simulink model "VTOLAutopilotController"  (R2025a)
settings: configuration reference "VTOLConfiguration" (kept outside this file)
undefined symbols (not defined in the file): Back_Transition_Rate, const, control, controlParams, ControlSampleTime, CriticalTiltAngle, DiscIntNeverNeededParam, dspblkCoreblockFVToolHelper, Fading_time, flightState, FSState, FWControlParams, FWTrimSpeed, gcbh, HoverMission, ReferenceFilterDen, ReferenceFilterNum, tilt_max, tiltIni, TransitioncontrolGains, uavParam, uavParams, VTOLcontrolGains, w_trim, WindDownRate
libraries: simulink x43, slpidlib x35, uavalgslib x7, simulink_extras x1
(part 4 of 8)

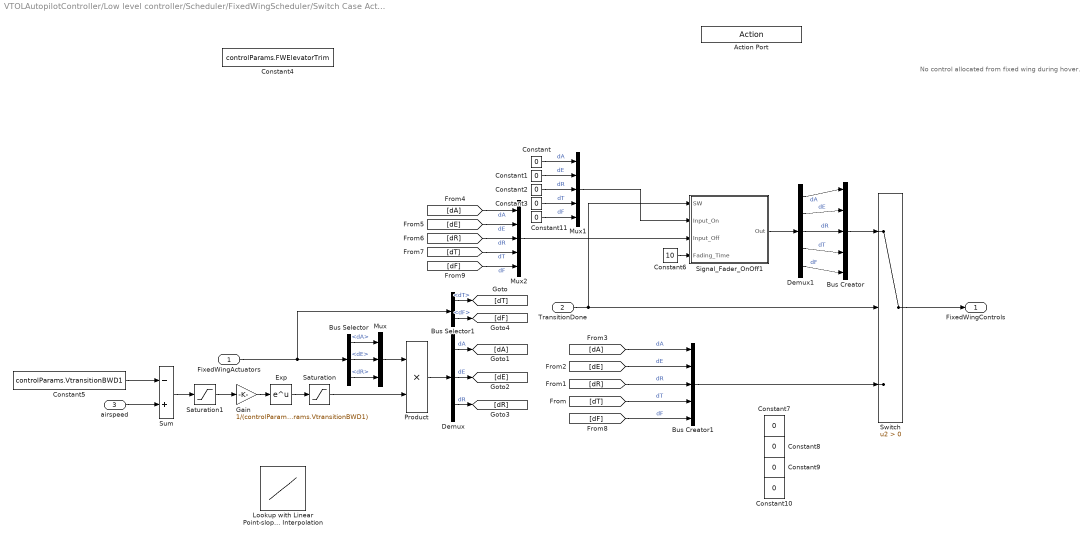
== system VTOLAutopilotController/Low level controller/Scheduler/FixedWingScheduler/Switch Case Action Subsystem3 ==
  note: No control allocated from fixed wing during hover.
  FixedWingActuators : Inport  OutDataTypeStr=Bus: FixedWingCtrlBus
  TransitionDone : Inport  Port=2
  airspeed : Inport  Port=3
  Action Port : ActionPort  ActionPortLabel=case [ BackTransition ]:
  Bus Creator : BusCreator  Inputs=5
  Bus Creator1 : BusCreator  Inputs=5  OutDataTypeStr=Bus: FixedWingCtrlBus
  Bus Selector : BusSelector  OutputSignals=dA,dE,dR
  Bus Selector1 : BusSelector  OutputSignals=dT,dF
  Constant{,1..3,7..11} (9 alike) : Constant  Value=0
  Constant4 : Constant  Value=controlParams.FWElevatorTrim
  Constant5 : Constant  Value=controlParams.VtransitionBWD1
  Constant6 : Constant  Value=10
  Demux : Demux  Outputs=3
  Demux1 : Demux  Outputs=5
  Exp : Math
  Gain : Gain  Gain=1/(controlParams.VtransitionBWD2-controlParams.VtransitionBWD1)
  Lookup with Linear Point-slope Interpolation : Lookup_n-D  NumberOfTableDimensions=1  BreakpointsForDimension1=[10 20 30 40 50 60]*const.kts2mps  Table=[1.0 1.0 0.8 0.5 0.1]  InternalRulePriority=Speed  RndMeth=Simplest
  Mux : Mux  Inputs=3
  Mux1 : Mux  Inputs=5
  Mux2 : Mux  Inputs=5
  Product : Product
  Saturation : Saturate  UpperLimit=1  LowerLimit=0
  Saturation1 : Saturate  UpperLimit=0  LowerLimit=controlParams.VtransitionBWD2-controlParams.VtransitionBWD1
  Signal_Fader_OnOff1 : Subsystem
  Sum : Sum  Inputs=-+
  Switch : Switch  Criteria=u2 > Threshold  SaturateOnIntegerOverflow=off  InputSameDT=off
  FixedWingControls : Outport  OutDataTypeStr=Bus: FixedWingCtrlBus
  wires:
  Bus Selector1/1 -> [dT]  "<dT>"
  Saturation1/1 -> Gain/1
  Demux/2 -> [dE]  "dE"
  Mux/1 -> Product/1
  Bus Selector/1 -> Mux/1  "<dA>"
  Bus Selector/2 -> Mux/2  "<dE>"
  Sum/1 -> Saturation1/1
  Product/1 -> Demux/1
  Constant5/1 -> Sum/1
  Saturation/1 -> Product/2
  Exp/1 -> Saturation/1
  Bus Selector/3 -> Mux/3  "<dR>"
  TransitionDone/1 -> Signal_Fader_OnOff1/1(SW), Switch/2
  FixedWingActuators/1 -> Bus Selector1/1, Bus Selector/1
  Demux/1 -> [dA]  "dA"
  airspeed/1 -> Sum/2
  Demux/3 -> [dR]  "dR"
  Gain/1 -> Exp/1
  Switch/1 -> FixedWingControls/1
  Constant6/1 -> Signal_Fader_OnOff1/4(Fading_Time)
  Bus Creator/1 -> Switch/1
  Demux1/3 -> Bus Creator/3  "dR"
  Demux1/2 -> Bus Creator/2  "dE"
  Demux1/4 -> Bus Creator/4  "dT"
  Demux1/1 -> Bus Creator/1  "dA"
  Signal_Fader_OnOff1/1(Out) -> Demux1/1
  Constant/1 -> Mux1/1  "dA"
  Constant1/1 -> Mux1/2  "dE"
  Constant2/1 -> Mux1/3  "dR"
  Constant3/1 -> Mux1/4  "dT"
  [dA] -> Mux2/1  "dA"
  [dE] -> Mux2/2  "dE"
  [dR] -> Mux2/3  "dR"
  [dT] -> Mux2/4  "dT"
  Mux1/1 -> Signal_Fader_OnOff1/2(Input_On)
  Mux2/1 -> Signal_Fader_OnOff1/3(Input_Off)
  Bus Creator1/1 -> Switch/3
  [dA] -> Bus Creator1/1  "dA"
  [dE] -> Bus Creator1/2  "dE"
  [dR] -> Bus Creator1/3  "dR"
  [dT] -> Bus Creator1/4  "dT"
  Constant11/1 -> Mux1/5  "dF"
  Bus Selector1/2 -> [dF]  "<dF>"
  [dF] -> Mux2/5  "dF"
  Demux1/5 -> Bus Creator/5  "dF"
  [dF] -> Bus Creator1/5  "dF"

== system VTOLAutopilotController/Low level controller/Scheduler/Subsystem/Actuator To Voltage ==
  note: #2, 25/05/20, MH, Fixed
      | The rotor rotational speed command should be
      | normalized to [rad/s].Previously, division by 2PI
      | was omitted in the command block,
      | while the 'Rotor Assembly' block multiplies
      | the input by 2PI, leading to increased gains.
  Motor Commands : Inport
  Bus Creator : BusCreator  Inputs=6  OutDataTypeStr=Bus: RotorCtrlBus
  Bus Selector : BusSelector  OutputSignals=w1,w2,w3,w4,Tilt1,Tilt2
  Gain{,1..2,4} (4 alike) : Gain  Gain=1/(uavParams.motor.RPMMAX/60)
  Gain3 : Gain  Gain=1/(pi/2)
  Gain5 : Gain  Gain=1/(pi/2)
  Gain{6..9} (4 alike) : Gain  Gain=1/(2*pi)
  Saturation{,1..3} (4 alike) : Saturate  UpperLimit=controlParams.maxPWM  LowerLimit=controlParams.minPWM
  Saturation4 : Saturate  UpperLimit=1  LowerLimit=0
  Saturation5 : Saturate  UpperLimit=1  LowerLimit=0
  To PWM : Outport
  wires:
  Motor Commands/1 -> Bus Selector/1
  Bus Selector/1 -> Gain/1  "<w1>"
  Bus Selector/3 -> Gain1/1  "<w3>"
  Bus Selector/2 -> Gain4/1  "<w2>"
  Bus Selector/4 -> Gain2/1  "<w4>"
  Bus Selector/5 -> Gain3/1  "<Tilt1>"
  Bus Selector/6 -> Gain5/1  "<Tilt2>"
  Gain/1 -> Gain6/1  "w1"
  Gain4/1 -> Gain7/1  "w2"
  Gain1/1 -> Gain8/1  "w3"
  Gain2/1 -> Gain9/1  "w4"
  Gain3/1 -> Saturation4/1
  Gain5/1 -> Saturation5/1
  Bus Creator/1 -> To PWM/1
  Gain6/1 -> Saturation/1
  Gain7/1 -> Saturation1/1
  Gain8/1 -> Saturation2/1
  Gain9/1 -> Saturation3/1
  Saturation/1 -> Bus Creator/1  "w1"
  Saturation1/1 -> Bus Creator/2  "w2"
  Saturation2/1 -> Bus Creator/3  "w3"
  Saturation3/1 -> Bus Creator/4  "w4"
  Saturation4/1 -> Bus Creator/5  "Tilt1"
  Saturation5/1 -> Bus Creator/6  "Tilt2"

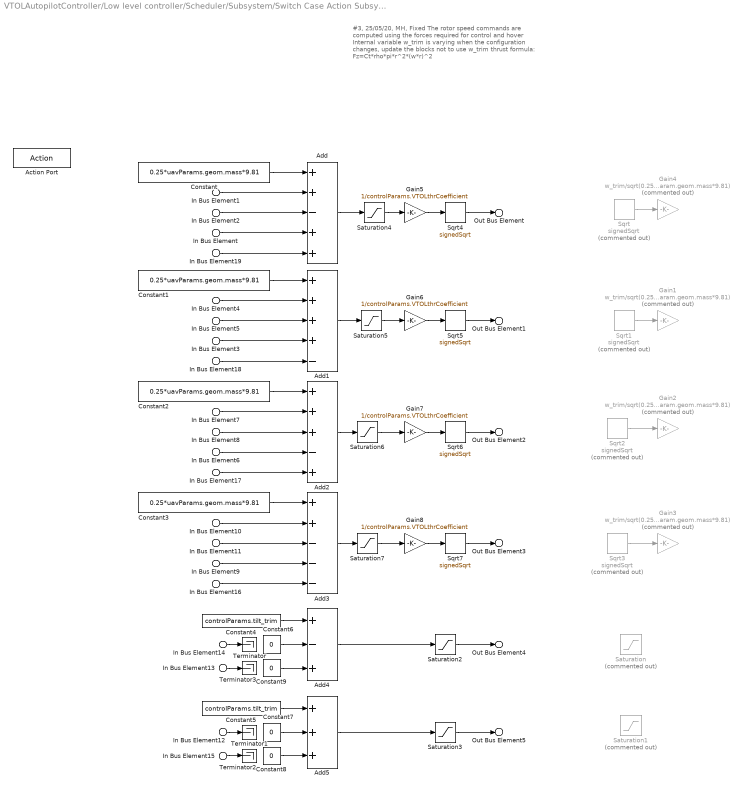
== system VTOLAutopilotController/Low level controller/Scheduler/Subsystem/Switch Case Action Subsystem ==
  note: #3, 25/05/20, MH, Fixed
      | The rotor speed commands are computed using
      | the forces required for control and hover
      | Internal variable w_trim is varying when the
      | configuration changes, update the blocks not to
      | use w_trim
      | thrust formula: Fz=Ct*rho*pi*r^2*(w*r)^2
  In Bus Element{,3,6,9} (4 alike) : Inport  PortName=MixerCommands  Element=w_theta
  In Bus Element{1,4,7,10} (4 alike) : Inport  PortName=MixerCommands  Element=w_z
  In Bus Element{2,5,8,11} (4 alike) : Inport  PortName=MixerCommands  Element=w_phi
  In Bus Element{12,14,16..19} (6 alike) : Inport  PortName=MixerCommands  Element=w_psi
  In Bus Element13 : Inport  PortName=MixerCommands  Element=w_tilt
  In Bus Element15 : Inport  PortName=MixerCommands  Element=w_tilt
  Action Port : ActionPort  ActionPortLabel=case [ Hover ]:
  Add : Sum  Inputs=++-++
  Add1 : Sum  Inputs=++++-
  Add2 : Sum  Inputs=+++-+
  Add3 : Sum  Inputs=++---
  Add4 : Sum  Inputs=+-+
  Add5 : Sum  Inputs=+++
  Constant{,1..3} (4 alike) : Constant  Value=0.25*uavParams.geom.mass*9.81
  Constant4 : Constant  Value=controlParams.tilt_trim
  Constant5 : Constant  Value=controlParams.tilt_trim
  Constant{6..9} (4 alike) : Constant  Value=0
  Gain{1..4} (4 alike) : Gain  Commented=on  Gain=w_trim/sqrt(0.25*uavParam.geom.mass*9.81)
  Gain{5..8} (4 alike) : Gain  Gain=1/controlParams.VTOLthrCoefficient
  Saturation : Saturate  Commented=on  UpperLimit=tilt_max  LowerLimit=-tilt_max
  Saturation1 : Saturate  Commented=on  UpperLimit=tilt_max  LowerLimit=-tilt_max
  Saturation2 : Saturate  UpperLimit=tilt_max  LowerLimit=-tilt_max
  Saturation3 : Saturate  UpperLimit=tilt_max  LowerLimit=-tilt_max
  Saturation{4..7} (4 alike) : Saturate  UpperLimit=inf  LowerLimit=0
  Sqrt{,1..3} (4 alike) : Sqrt  Commented=on  Operator=signedSqrt
  Sqrt{4..7} (4 alike) : Sqrt  Operator=signedSqrt
  Terminator{,1..3} (4 alike) : Terminator
  Out Bus Element : Outport  PortName=Actuator  Element=w1
  Out Bus Element1 : Outport  PortName=Actuator  Element=w2
  Out Bus Element2 : Outport  PortName=Actuator  Element=w3
  Out Bus Element3 : Outport  PortName=Actuator  Element=w4
  Out Bus Element4 : Outport  PortName=Actuator  Element=Tilt1
  Out Bus Element5 : Outport  PortName=Actuator  Element=Tilt2
  wires:
  Constant5/1 -> Add5/1
  Constant2/1 -> Add2/1
  Constant1/1 -> Add1/1
  Constant4/1 -> Add4/1
  Constant/1 -> Add/1
  Constant3/1 -> Add3/1
  Add/1 -> Saturation4/1
  Add1/1 -> Saturation5/1
  Add2/1 -> Saturation6/1
  Add3/1 -> Saturation7/1
  Saturation2/1 -> Out Bus Element4/1
  Add4/1 -> Saturation2/1
  Add5/1 -> Saturation3/1
  Saturation3/1 -> Out Bus Element5/1
  Saturation4/1 -> Gain5/1
  Saturation5/1 -> Gain6/1
  Saturation6/1 -> Gain7/1
  Saturation7/1 -> Gain8/1
  Sqrt4/1 -> Out Bus Element/1
  Sqrt5/1 -> Out Bus Element1/1
  Sqrt6/1 -> Out Bus Element2/1
  Sqrt7/1 -> Out Bus Element3/1
  In Bus Element2/1 -> Add/3
  In Bus Element/1 -> Add/4
  In Bus Element5/1 -> Add1/3
  In Bus Element3/1 -> Add1/4
  In Bus Element8/1 -> Add2/3
  In Bus Element11/1 -> Add3/3
  In Bus Element9/1 -> Add3/4
  In Bus Element6/1 -> Add2/4
  Sqrt/1 -> Gain4/1
  Sqrt3/1 -> Gain3/1
  Sqrt2/1 -> Gain2/1
  Sqrt1/1 -> Gain1/1
  Gain5/1 -> Sqrt4/1
  Gain6/1 -> Sqrt5/1
  Gain7/1 -> Sqrt6/1
  Gain8/1 -> Sqrt7/1
  In Bus Element1/1 -> Add/2
  In Bus Element4/1 -> Add1/2
  In Bus Element7/1 -> Add2/2
  In Bus Element10/1 -> Add3/2
  In Bus Element19/1 -> Add/5
  In Bus Element16/1 -> Add3/5
  In Bus Element17/1 -> Add2/5
  In Bus Element18/1 -> Add1/5
  In Bus Element14/1 -> Terminator/1
  In Bus Element12/1 -> Terminator1/1
  Constant6/1 -> Add4/2
  Constant7/1 -> Add5/2
  Constant8/1 -> Add5/3
  In Bus Element15/1 -> Terminator2/1
  Constant9/1 -> Add4/3
  In Bus Element13/1 -> Terminator3/1

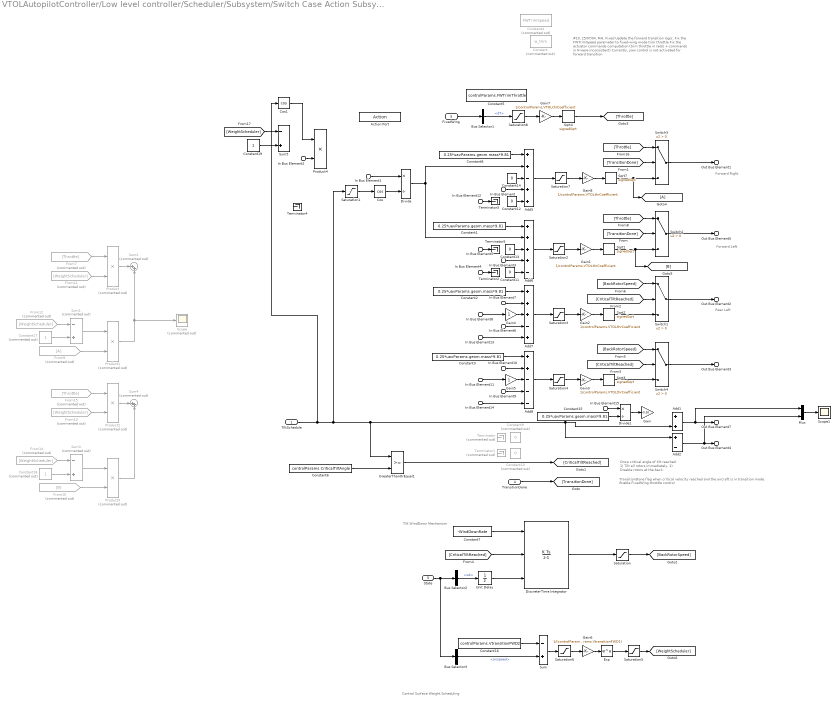
== system VTOLAutopilotController/Low level controller/Scheduler/Subsystem/Switch Case Action Subsystem1 ==
  note: Tilt WindDown Mechanism
  note: Once critical angle of tilt reached.
      | 1) Tilt all rotors immediately.
      | 2) Disable rotors at the back.
  note: TransitionDone flag when critical velocity reached and the aircraft is in transition mode.
      | Enable FixedWing throttle control
  note: #10, 25/07/04, MH, Fixed
      | Update the forward transition logic.
      | Fix the FWTrimSpeed parameter to fixed-wing
      | mode trim throttle
      | Fix the actuator commands computation
      | (trim throttle in rad/s + commands in N were
      | inconsistent)
      | Currently, yaw control is not activated for
      | forward transition
  note: Rear Left
  note: Forward Right
  note: Forward Left
  note: Control Surface Weight Scheduling
  TiltSchedule : Inport
  In Bus Element{,3,6,9} (4 alike) : Inport  Port=2  PortName=MixerCommands  Element=w_theta
  In Bus Element1 : Inport  Port=2  PortName=MixerCommands  Element=w_z
  In Bus Element7 : Inport  Port=2  PortName=MixerCommands  Element=w_z
  In Bus Element10 : Inport  Port=2  PortName=MixerCommands  Element=w_z
  In Bus Element{2,5,8,11} (4 alike) : Inport  Port=2  PortName=MixerCommands  Element=w_phi
  In Bus Element{4,12..15} (5 alike) : Inport  Port=2  PortName=MixerCommands  Element=w_psi
  FixedWing : Inport  Port=3
  TransitionDone : Inport  Port=4
  State : Inport  Port=5
  Action Port : ActionPort  ActionPortLabel=case [ Transition ]:
  Add1 : Sum
  Add2 : Sum  Inputs=+-
  Add5 : Sum  Inputs=++-++
  Add6 : Sum  Inputs=++++-
  Add7 : Sum  Inputs=+++-+
  Add8 : Sum  Inputs=++---
  Bus Selector1 : BusSelector  OutputSignals=dT
  Bus Selector2 : BusSelector  OutputSignals=RotorParameters.w4
  Bus Selector3 : BusSelector  OutputSignals=airspeed
  Constant : Constant  Commented=on  Value=w_trim
  Constant{1..3,8,15} (5 alike) : Constant  Value=0.25*uavParams.geom.mass*9.81
  Constant10 : Constant  Commented=on  Value=0
  Constant{11..14} (4 alike) : Constant  Value=0
  Constant16 : Constant  Value=controlParams.VtransitionFWD2
  Constant17 : Constant  Commented=on
  Constant18 : Constant  Commented=on
  Constant19 : Constant
  Constant4 : Constant  Commented=on  Value=FWTrimSpeed
  Constant5 : Constant  Value=controlParams.FWTrimThrottle
  Constant6 : Constant  Value=controlParams.CriticalTiltAngle
  Constant7 : Constant  Value=-WindDownRate
  Constant9 : Constant  Commented=on  Value=0
  Cos : Trigonometry  Operator=cos
  Cos1 : Trigonometry  Operator=cos
  Discrete-Time Integrator : DiscreteIntegrator  ExternalReset=either  InitialConditionSource=external  SampleTime=0.005  ICPrevOutput=DiscIntNeverNeededParam  ICPrevScaledInput=DiscIntNeverNeededParam
  Divide : Product  Inputs=*/
  Divide1 : Product  Inputs=*/
  Exp : Math
  From10 : From  Commented=on  GotoTag=B
  From{11..14} (4 alike) : From  Commented=on  GotoTag=WeightScheduler
  From15 : From  Commented=on  GotoTag=Throttle
  From7 : From  Commented=on  GotoTag=Throttle
  From9 : From  Commented=on
  Gain : Gain  Gain=-0.30
  Gain{1..3,7..8} (5 alike) : Gain  Gain=1/controlParams.VTOLthrCoefficient
  Gain4 : Gain
  Gain5 : Gain
  Gain6 : Gain  Gain=1/(controlParams.VtransitionFWD2-controlParams.VtransitionFWD1)
  Goto4 : Goto
  GreaterThanOrEqual1 : RelationalOperator  OutDataTypeStr=boolean  RndMeth=Simplest  InputSameDT=off
  Mux : Mux  Inputs=2
  Product{,1..3} (4 alike) : Product  Commented=on
  Product4 : Product
  Saturation : Saturate  UpperLimit=Inf  LowerLimit=0
  Saturation1 : Saturate  UpperLimit=CriticalTiltAngle  LowerLimit=-CriticalTiltAngle
  Saturation{2..4,7..8} (5 alike) : Saturate  UpperLimit=inf  LowerLimit=0
  Saturation5 : Saturate  UpperLimit=1  LowerLimit=0
  Saturation6 : Saturate  UpperLimit=0  LowerLimit=controlParams.VtransitionFWD1-controlParams.VtransitionFWD2
  Scope : Scope  Commented=on
      settings: ActiveDisplayYMinimum=-118.86543  ActiveDisplayYMaximum=1069.7889
  Scope1 : Scope
      settings: ActiveDisplayYMinimum=-0.19635  ActiveDisplayYMaximum=1.76715  DataLoggingVariableName=ScopeData3
  Sqrt{1..4,7} (5 alike) : Sqrt  Operator=signedSqrt
  Sum : Sum  Inputs=-+
  Sum1 : Sum  Commented=on  Inputs=-+
  Sum2 : Sum  Commented=on  Inputs=|++
  Sum3 : Sum  Commented=on  Inputs=-+
  Sum4 : Sum  Commented=on  Inputs=|++
  Sum5 : Sum  Inputs=-+
  Switch{1..4} (4 alike) : Switch  Criteria=u2 > Threshold  SaturateOnIntegerOverflow=off  InputSameDT=off
  Terminator : Terminator  Commented=on
  Terminator1 : Terminator  Commented=on
  Terminator{2..5} (4 alike) : Terminator
  Unit Delay : UnitDelay  SampleTime=-1  HasFrameUpgradeWarning=on
  Out Bus Element1 : Outport  PortName=Actuator  Element=w1
  Out Bus Element5 : Outport  PortName=Actuator  Element=w2
  Out Bus Element2 : Outport  PortName=Actuator  Element=w3
  Out Bus Element3 : Outport  PortName=Actuator  Element=w4
  Out Bus Element7 : Outport  PortName=Actuator  Element=Tilt1
  Out Bus Element4 : Outport  PortName=Actuator  Element=Tilt2
  wires:
  TiltSchedule/1 -> Cos1/1, GreaterThanOrEqual1/1, Add2/1, Add1/2, Saturation1/1
  In Bus Element9/1 -> Add8/4
  In Bus Element6/1 -> Add7/4
  Constant3/1 -> Add8/1
  In Bus Element/1 -> Add5/4
  In Bus Element10/1 -> Add8/2
  Constant1/1 -> Add6/1
  In Bus Element3/1 -> Add6/4
  In Bus Element7/1 -> Add7/2
  Constant2/1 -> Add7/1
  FixedWing/1 -> Bus Selector1/1
  [TransitionDone] -> Switch3/2
  Constant6/1 -> GreaterThanOrEqual1/2
  GreaterThanOrEqual1/1 -> [CriticalTiltReached]
  [CriticalTiltReached] -> Switch1/2
  [CriticalTiltReached] -> Switch4/2
  TransitionDone/1 -> [TransitionDone]
  Bus Selector2/1 -> Unit Delay/1  "<w4>"
  Constant7/1 -> Discrete-Time Integrator/1
  [CriticalTiltReached] -> Discrete-Time Integrator/2
  Discrete-Time Integrator/1 -> Saturation/1
  Saturation/1 -> [BackRotorSpeed]
  State/1 -> Bus Selector3/1, Bus Selector2/1
  Unit Delay/1 -> Discrete-Time Integrator/3
  Cos/1 -> Divide/2
  Saturation1/1 -> Cos/1
  In Bus Element1/1 -> Divide/1
  Divide/1 -> Add5/2, Add6/2
  Switch1/1 -> Out Bus Element2/1
  Gain8/1 -> Sqrt7/1
  Saturation7/1 -> Gain8/1
  Constant8/1 -> Add5/1
  Add5/1 -> Saturation7/1
  Sqrt7/1 -> Goto4/1, Switch3/3
  [TransitionDone] -> Switch2/2
  Saturation2/1 -> Gain1/1
  Gain1/1 -> Sqrt1/1
  Add6/1 -> Saturation2/1
  Sqrt1/1 -> [B], Switch2/3
  Gain2/1 -> Sqrt2/1
  Saturation3/1 -> Gain2/1
  Add7/1 -> Saturation3/1
  Gain3/1 -> Sqrt3/1
  Saturation4/1 -> Gain3/1
  Add8/1 -> Saturation4/1
  Constant11/1 -> Add6/5
  Constant12/1 -> Add5/5
  In Bus Element12/1 -> Terminator3/1
  In Bus Element4/1 -> Terminator2/1
  Sqrt3/1 -> Switch4/3
  Switch4/1 -> Out Bus Element3/1
  Sqrt2/1 -> Switch1/3
  [BackRotorSpeed] -> Switch1/1
  [BackRotorSpeed] -> Switch4/1
  In Bus Element2/1 -> Product4/2
  In Bus Element5/1 -> Terminator5/1
  In Bus Element11/1 -> Gain5/1
  In Bus Element8/1 -> Gain4/1
  Add1/1 -> Mux/1, Out Bus Element7/1
  In Bus Element13/1 -> Add7/5
  In Bus Element14/1 -> Add8/5
  In Bus Element15/1 -> Divide1/1
  Constant15/1 -> Divide1/2
  Divide1/1 -> Gain/1
  Add2/1 -> Mux/2, Out Bus Element4/1
  Gain4/1 -> Add7/3
  Gain5/1 -> Add8/3
  Saturation6/1 -> Gain6/1
  Sum/1 -> Saturation6/1
  Product/1 -> Sum2/1
  Constant16/1 -> Sum/1
  Gain6/1 -> Exp/1
  Exp/1 -> Saturation5/1
  From7/1 -> Product/1
  Constant17/1 -> Sum1/2
  Sum1/1 -> Product1/1
  From9/1 -> Product1/2
  Product1/1 -> Scope/1, Sum2/2
  [Throttle] -> Switch2/1
  Saturation5/1 -> [WeightScheduler]
  From11/1 -> Product/2
  From12/1 -> Sum1/1
  Product3/1 -> Sum4/2
  From14/1 -> Sum3/1
  Constant18/1 -> Sum3/2
  Product2/1 -> Sum4/1
  Sum3/1 -> Product3/1
  From10/1 -> Product3/2
  From15/1 -> Product2/1
  From13/1 -> Product2/2
  [Throttle] -> Switch3/1
  Bus Selector3/1 -> Sum/2  "<airspeed>"
  Switch3/1 -> Out Bus Element1/1
  Switch2/1 -> Out Bus Element5/1
  Mux/1 -> Scope1/1
  Constant19/1 -> Sum5/2
  [WeightScheduler] -> Sum5/1
  Cos1/1 -> Product4/1
  Constant13/1 -> Add6/3
  Constant14/1 -> Add5/3
  Saturation8/1 -> Gain7/1
  Gain7/1 -> Sqrt4/1
  Bus Selector1/1 -> Saturation8/1  "<dT>"
  Sqrt4/1 -> [Throttle]

== system VTOLAutopilotController/Low level controller/Scheduler/Subsystem/Switch Case Action Subsystem2 ==
  note: Tilt WindDown Mechanism
  In Bus Element2 : Inport  PortName=FixedWingCtrlBus  Element=dT
  In Bus Element1 : Inport  PortName=FixedWingCtrlBus  Element=dT
  TransitionDone : Inport  Port=2
  State : Inport  Port=3
  Action Port : ActionPort  ActionPortLabel=case [ FixedWing ]:
  Add : Sum  Commented=on
  Add1 : Sum  Commented=on
  Bus Selector2 : BusSelector  OutputSignals=RotorParameters.w4
  Constant : Constant  Commented=on  Value=FWTrimSpeed
  Constant1 : Constant  Value=-WindDownRate
  Constant4 : Constant  Value=pi/2
  Constant5 : Constant  Commented=on  Value=controlParams.FWTrimThrottle
  Constant7 : Constant  Value=pi/2
  Discrete-Time Integrator : DiscreteIntegrator  ExternalReset=rising  InitialConditionSource=external  SampleTime=0.005  ICPrevOutput=DiscIntNeverNeededParam  ICPrevScaledInput=DiscIntNeverNeededParam
  Gain1 : Gain  Gain=1/controlParams.VTOLthrCoefficient
  Gain7 : Gain  Gain=1/controlParams.VTOLthrCoefficient
  Saturation : Saturate  UpperLimit=Inf  LowerLimit=0
  Saturation1 : Saturate  UpperLimit=Inf  LowerLimit=0
  Saturation2 : Saturate  UpperLimit=Inf  LowerLimit=0
  Saturation3 : Saturate  UpperLimit=inf  LowerLimit=0
  Saturation8 : Saturate  UpperLimit=inf  LowerLimit=0
  Sqrt1 : Sqrt  Operator=signedSqrt
  Sqrt4 : Sqrt  Operator=signedSqrt
  Out Bus Element : Outport  PortName=Actuator  Element=w1
  Out Bus Element1 : Outport  PortName=Actuator  Element=w2
  Out Bus Element2 : Outport  PortName=Actuator  Element=w3
  Out Bus Element3 : Outport  PortName=Actuator  Element=w4
  Out Bus Element7 : Outport  PortName=Actuator  Element=Tilt1
  Out Bus Element4 : Outport  PortName=Actuator  Element=Tilt2
  wires:
  Sqrt1/1 -> Saturation1/1
  Constant4/1 -> Out Bus Element4/1
  [BackRotorSpeed] -> Out Bus Element2/1
  Constant7/1 -> Out Bus Element7/1
  In Bus Element2/1 -> Saturation3/1
  Sqrt4/1 -> Saturation/1
  In Bus Element1/1 -> Saturation8/1
  Saturation/1 -> Out Bus Element/1
  Saturation1/1 -> Out Bus Element1/1
  [BackRotorSpeed] -> Out Bus Element3/1
  Bus Selector2/1 -> Discrete-Time Integrator/3  "<w4>"
  Saturation2/1 -> [BackRotorSpeed]
  State/1 -> Bus Selector2/1
  Constant1/1 -> Discrete-Time Integrator/1
  Discrete-Time Integrator/1 -> Saturation2/1
  TransitionDone/1 -> Discrete-Time Integrator/2
  Saturation8/1 -> Gain7/1
  Gain7/1 -> Sqrt4/1
  Saturation3/1 -> Gain1/1
  Gain1/1 -> Sqrt1/1

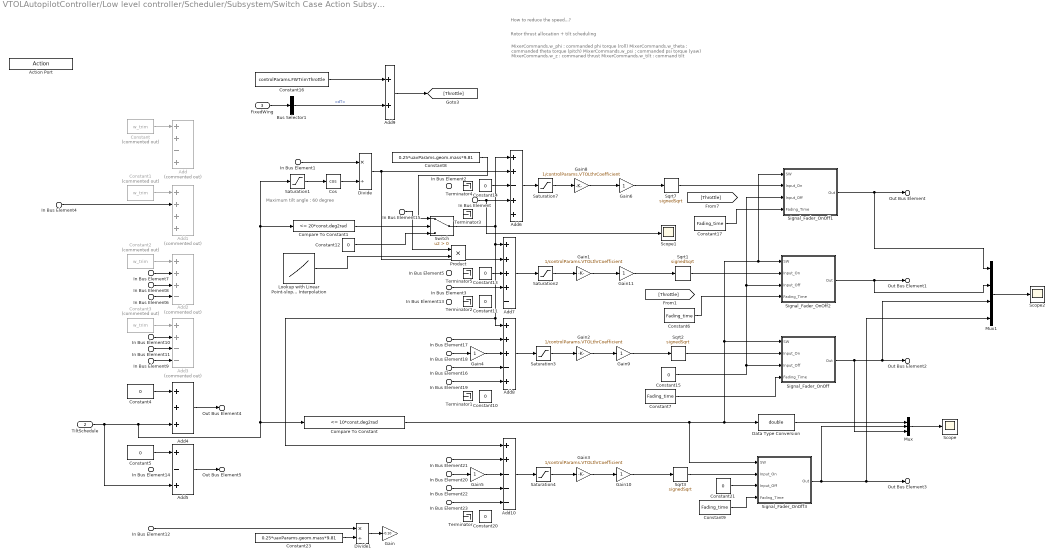
== system VTOLAutopilotController/Low level controller/Scheduler/Subsystem/Switch Case Action Subsystem3 ==
  note: Maximum tilt angle : 60 degree
  note: MixerCommands.w_phi : commanded phi torque (roll)
      | MixerCommands.w_theta : commanded theta torque (pitch)
      | MixerCommands.w_psi : commanded psi torque (yaw)
      | MixerCommands.w_z : commaned thrust
      | MixerCommands.w_tilt : command tilt
  note: Rotor thrust allocation + tilt scheduling
  note: How to reduce the speed...?
  In Bus Element{,3,6,9,16,22} (6 alike) : Inport  PortName=MixerCommands  Element=w_theta
  In Bus Element{1,4,7,10,17,21} (6 alike) : Inport  PortName=MixerCommands  Element=w_z
  In Bus Element{2,5,8,11,18,20} (6 alike) : Inport  PortName=MixerCommands  Element=w_phi
  In Bus Element{12..15,19,23} (6 alike) : Inport  PortName=MixerCommands  Element=w_psi
  TiltSchedule : Inport  Port=2
  FixedWing : Inport  Port=3
  Action Port : ActionPort  ActionPortLabel=case [ BackTransition ]:
  Add : Sum  Commented=on  Inputs=++-+
  Add1 : Sum  Commented=on  Inputs=++++
  Add10 : Sum  Inputs=++---
  Add2 : Sum  Commented=on  Inputs=+++-
  Add3 : Sum  Commented=on  Inputs=++--
  Add4 : Sum  Inputs=+++
  Add5 : Sum  Inputs=+-+
  Add6 : Sum  Inputs=++-++
  Add7 : Sum  Inputs=++++-
  Add8 : Sum  Inputs=+++-+
  Add9 : Sum
  Bus Selector1 : BusSelector  OutputSignals=dT
  Compare To Constant : simulink/Logic and Bit Operations/Compare To Constant  relop=<=  const=10*const.deg2rad  OutDataTypeStr=boolean
  Compare To Constant1 : simulink/Logic and Bit Operations/Compare To Constant  relop=<=  const=20*const.deg2rad  OutDataTypeStr=boolean
  Constant{,1..3} (4 alike) : Constant  Commented=on  Value=w_trim
  Constant{4..5,10..15,20..21} (10 alike) : Constant  Value=0
  Constant16 : Constant  Value=controlParams.FWTrimThrottle
  Constant{6..7,9,17} (4 alike) : Constant  Value=Fading_time
  Constant23 : Constant  Value=0.25*uavParams.geom.mass*9.81
  Constant8 : Constant  Value=0.25*uavParams.geom.mass*9.81
  Cos : Trigonometry  Operator=cos
  Data Type Conversion : DataTypeConversion  OutDataTypeStr=double  SaturateOnIntegerOverflow=off  RndMeth=Floor
  Divide : Product  Inputs=*/
  Divide1 : Product  Inputs=*/
  Gain : Gain  Gain=-0.10
  Gain{1..3,8} (4 alike) : Gain  Gain=1/controlParams.VTOLthrCoefficient
  Gain{4..6,9..11} (6 alike) : Gain
  Lookup with Linear Point-slope Interpolation : Lookup_n-D  NumberOfTableDimensions=1  BreakpointsForDimension1=[10 20 30 40 50 60]*const.kts2mps  Table=[1.0 1.0 0.8 0.5 0.1]  InternalRulePriority=Speed  RndMeth=Simplest
  Mux : Mux  Inputs=3
  Mux1 : Mux
  Product : Product
  Saturation1 : Saturate  UpperLimit=controlParams.CriticalTiltAngle  LowerLimit=-controlParams.CriticalTiltAngle
  Saturation{2..4,7} (4 alike) : Saturate  UpperLimit=inf  LowerLimit=0
  Scope : Scope
      settings: ActiveDisplayYMinimum=-11.37479  ActiveDisplayYMaximum=68.93084  DataLoggingVariableName=ScopeData5
  Scope1 : Scope
      settings: ActiveDisplayYMinimum=-91.47313  ActiveDisplayYMaximum=823.25813
  Scope2 : Scope
      settings: ActiveDisplayYMinimum=325.4581  ActiveDisplayYMaximum=599.86957  DataLoggingVariableName=ScopeData2
  Signal_Fader_OnOff : Subsystem
  Signal_Fader_OnOff1 : Subsystem
  Signal_Fader_OnOff2 : Subsystem
  Signal_Fader_OnOff3 : Subsystem
  Sqrt{1..3,7} (4 alike) : Sqrt  Operator=signedSqrt
  Switch : Switch  Criteria=u2 > Threshold  SaturateOnIntegerOverflow=off  InputSameDT=off
  Terminator{,1..5} (6 alike) : Terminator
  Out Bus Element : Outport  PortName=Actuator  Element=w1
  Out Bus Element1 : Outport  PortName=Actuator  Element=w2
  Out Bus Element2 : Outport  PortName=Actuator  Element=w3
  Out Bus Element3 : Outport  PortName=Actuator  Element=w4
  Out Bus Element4 : Outport  PortName=Actuator  Element=Tilt1
  Out Bus Element5 : Outport  PortName=Actuator  Element=Tilt2
  wires:
  In Bus Element4/1 -> Add1/2
  In Bus Element11/1 -> Add3/3
  In Bus Element8/1 -> Add2/3
  Constant2/1 -> Add2/1
  In Bus Element9/1 -> Add3/4
  In Bus Element6/1 -> Add2/4
  Constant1/1 -> Add1/1
  In Bus Element10/1 -> Add3/2
  Constant/1 -> Add/1
  Constant3/1 -> Add3/1
  In Bus Element7/1 -> Add2/2
  Constant4/1 -> Add4/1
  Constant5/1 -> Add5/1
  Add4/1 -> Out Bus Element4/1
  Add5/1 -> Out Bus Element5/1
  Add6/1 -> Saturation7/1
  Signal_Fader_OnOff1/1(Out) -> Out Bus Element/1, Mux1/1
  Constant8/1 -> Switch/1
  In Bus Element/1 -> Scope1/1, Add6/4
  Saturation7/1 -> Gain8/1
  Gain8/1 -> Gain6/1
  Sqrt7/1 -> Signal_Fader_OnOff1/2(Input_On)
  Cos/1 -> Divide/2
  Saturation1/1 -> Cos/1
  In Bus Element1/1 -> Divide/1
  TiltSchedule/1 -> Add5/3, Add4/3, Compare To Constant/1, Saturation1/1, Compare To Constant1/1
  In Bus Element17/1 -> Add8/2
  Saturation2/1 -> Gain1/1
  Divide/1 -> Add7/2, Add6/2
  Sqrt1/1 -> Signal_Fader_OnOff2/2(Input_On)
  Saturation3/1 -> Gain2/1
  Sqrt2/1 -> Signal_Fader_OnOff/2(Input_On)
  Gain4/1 -> Add8/3
  Add8/1 -> Saturation3/1
  Gain1/1 -> Gain11/1
  Add7/1 -> Saturation2/1
  In Bus Element3/1 -> Add7/4
  Gain2/1 -> Gain9/1
  In Bus Element16/1 -> Add8/4
  In Bus Element18/1 -> Gain4/1
  Constant7/1 -> Signal_Fader_OnOff/4(Fading_Time)
  Constant15/1 -> Signal_Fader_OnOff1/3(Input_Off), Signal_Fader_OnOff2/3(Input_Off), Signal_Fader_OnOff/3(Input_Off)
  Constant16/1 -> Add9/1
  Add9/1 -> [Throttle]
  FixedWing/1 -> Bus Selector1/1
  Bus Selector1/1 -> Add9/2  "<dT>"
  Constant17/1 -> Signal_Fader_OnOff1/4(Fading_Time)
  Constant6/1 -> Signal_Fader_OnOff2/4(Fading_Time)
  Signal_Fader_OnOff2/1(Out) -> Mux1/2, Out Bus Element1/1
  Signal_Fader_OnOff/1(Out) -> Mux/3, Mux1/3, Out Bus Element2/1
  In Bus Element20/1 -> Gain5/1
  Add10/1 -> Saturation4/1
  Gain3/1 -> Gain10/1
  Sqrt3/1 -> Signal_Fader_OnOff3/2(Input_On)
  Saturation4/1 -> Gain3/1
  Gain5/1 -> Add10/3
  In Bus Element22/1 -> Add10/4
  In Bus Element21/1 -> Add10/2
  Constant9/1 -> Signal_Fader_OnOff3/4(Fading_Time)
  Constant21/1 -> Signal_Fader_OnOff3/3(Input_Off)
  Signal_Fader_OnOff3/1(Out) -> Mux/2, Out Bus Element3/1, Mux1/4
  Compare To Constant/1 -> Signal_Fader_OnOff3/1(SW), Signal_Fader_OnOff1/1(SW), Signal_Fader_OnOff2/1(SW), Signal_Fader_OnOff/1(SW), Data Type Conversion/1
  Mux/1 -> Scope/1
  Data Type Conversion/1 -> Mux/1
  Constant23/1 -> Divide1/2
  Divide1/1 -> Gain/1
  In Bus Element12/1 -> Divide1/1
  Constant13/1 -> Add7/3
  Constant14/1 -> Add6/3
  Compare To Constant1/1 -> Switch/2
  Constant12/1 -> Switch/3
  Switch/1 -> Add8/1, Add10/1, Add7/1, Add6/1
  In Bus Element19/1 -> Add8/5
  In Bus Element23/1 -> Add10/5
  Mux1/1 -> Scope2/1
  Gain6/1 -> Sqrt7/1
  Gain11/1 -> Sqrt1/1
  Gain9/1 -> Sqrt2/1
  Gain10/1 -> Sqrt3/1
  In Bus Element15/1 -> Product/1
  Lookup with Linear Point-slope Interpolation/1 -> Product/2

== system VTOLAutopilotController/Guidance Test Bench/ControlType/Guidance Testbench/Guidance Logic/Guidance Stateflow ==
  note: Can be replaced with a signal from the GCS to "Start Mission"
  Pose : Inport
  GCSCommands : Inport  Port=2
  LandingStates : Inport  Port=3
  States : Inport  Port=4
  Ground : Inport  Port=5
  "Bus " : BusSelector  Commented=on  OutputSignals=LAP,YawCmd
  Bus Selector : BusSelector  OutputSignals=mode
  Compare To Constant : simulink/Logic and Bit Operations/Compare To Constant  relop===  const=1  OutDataTypeStr=boolean
  Constant : Constant  Value=FSState
  Constant1 : Constant  Value=controlParams.VtransitionFWD1
  Constant2 : Constant  Value=controlParams.VtransitionFWD2
  Constant3 : Constant  Value=controlParams.PitchtransitionFWD
  Data Type Conversion : DataTypeConversion  OutDataTypeStr=uint8  SaturateOnIntegerOverflow=off  RndMeth=Floor
  Delay : Delay  DelayLength=1  InitialCondition=0
  Delay1 : Delay  DelayLength=1  InputProcessing=Columns as channels (frame based)
  Display : Display
  Guidance Mode Selector : Stateflow chart  TreatAsAtomicUnit=on  SystemSampleTime=0.02
      settings: PortSchema="{\"entries\":[{\"content\":{\"sides\":[{\"content\":{\"connectorIds\":[\"In1\",\"In2\",\"In3\",\"In4\",\"In5\",\"In6\",\"In7\",\"In8\",\"In9\",\"In10\"]},\"type\":\"ConnectorPlacement.EquallySpacedRectSide\",\"uuid\":\"a9cfd0e2-196c-422d-b359-9161a47768c9\"},{\"content\":{\"connectorIds\":[\"Out7\",\"Out8\",\"Out2\",\"Out3\",\"Out4\",\"Out5\",\"Out6\",\"Out1\"],\"side\":\"RIGHT\"},\"type\":\"ConnectorPlacement.EquallySpacedRectSide\",\"uuid\":\"4fed41ae-e7cf-4de3-8bdb-9e24e7d8b079\"},{\"content\":{\"side\":\"TOP\"},\"type\":\"ConnectorPlacement.EquallySpacedRectSide\",\"uuid\":\"2d49ff20-2f63-498d-ac9d-820eae01f794\"}]},\"type\":\"ConnectorPlacement.EquallySpacedConnector\",\"uuid\":\"88d403f4-ad96-40f9-9697-84906f26a8bf\"}],\"packageUris\":[\"http://schema.mathworks.com/mf0/Connector/R2020b\"],\"version\":\"1.0\"}"
  Home : Constant  Value=[0 0 0]  OutDataTypeStr=double
  Landed? : simulink/Logic and Bit Operations/Compare To Constant  relop===  const=2  OutDataTypeStr=boolean
  MissionAction : Constant  Value=0  OutDataTypeStr=uint8
  Mux : Mux  Commented=on  Inputs=2
  Rate Transition : RateTransition
  "Select \"From\" Waypoint" : Selector  InputPortWidth=2  IndexOptions=Index vector (dialog)  Indices=2  OutputSizes=1
  "Select \"To\" Waypoint" : Selector  InputPortWidth=2  IndexOptions=Index vector (dialog)  Indices=1  OutputSizes=1
  Stop Simulation : Stop
  Takeoff IC : InitialCondition
  UAV Path Manager : uavalgslib/Path Manager  UAVType=multirotor  LoiterRadius=25  dataType=double  inputBusName='doubleUavPathManager'  SimulateUsing=Code generation
  HoverSP : Outport
  VTOLSP : Outport  Port=2
  AACSP : Outport  Port=3
  FixedWingSP : Outport  Port=4
  CtrlMode : Outport  Port=5
  FlightMode : Outport  Port=6
  GuidanceMode : Outport  Port=7
  wires:
  Takeoff IC/1 -> Guidance Mode Selector/1(mode)
  MissionAction/1 -> UAV Path Manager/4
  Guidance Mode Selector/2(Status) -> Delay/1, Landed?/1
  Home/1 -> UAV Path Manager/5
  GCSCommands/1 -> UAV Path Manager/2
  UAV Path Manager/1 -> Rate Transition/1
  Bus Selector/1 -> Takeoff IC/1  "<mode>"
  [pose] -> Guidance Mode Selector/4(Pose)
  Compare To Constant/1 -> UAV Path Manager/3
  "Select \"To\" Waypoint"/1 -> Bus Selector/1, Guidance Mode Selector/2(ToWP)
  "Select \"From\" Waypoint"/1 -> Guidance Mode Selector/3(FromWP)
  Landed?/1 -> Stop Simulation/1
  Delay/1 -> Compare To Constant/1
  LandingStates/1 -> [landingState]
  States/1 -> Guidance Mode Selector/5(States)
  Guidance Mode Selector/5(ControlMode) -> CtrlMode/1
  Guidance Mode Selector/3(AACSP) -> AACSP/1
  Guidance Mode Selector/4(FixedWingSP) -> FixedWingSP/1
  Guidance Mode Selector/6(FlightMode) -> FlightMode/1, Data Type Conversion/1
  Constant/1 -> Guidance Mode Selector/6(PresetMode)
  Guidance Mode Selector/7(HoverSP) -> HoverSP/1
  Ground/1 -> Guidance Mode Selector/7(Ground)
  Pose/1 -> [pose], UAV Path Manager/1
  Rate Transition/1 -> "Select \"To\" Waypoint"/1, "Select \"From\" Waypoint"/1
  Constant1/1 -> Guidance Mode Selector/8(VFWDTransition1)
  Constant2/1 -> Guidance Mode Selector/9(VFWDTransition2)
  "Bus "/1 -> Mux/1  "<LAP>"
  "Bus "/2 -> Mux/2  "<YawCmd>"
  Guidance Mode Selector/1(GuidanceMode) -> GuidanceMode/1, Display/1
  Guidance Mode Selector/8(VTOLSP) -> VTOLSP/1
  Data Type Conversion/1 -> Delay1/1
  Delay1/1 -> Guidance Mode Selector/10(ModeFDBK)

== system VTOLAutopilotController/Guidance Test Bench/ControlType/Guidance Testbench/Guidance Logic/Interface ==
  UAVState : Inport
  Bus Creator : BusCreator  Inputs=5
  Bus Selector : BusSelector  OutputSignals=Xe,Ve
  Demux : Demux  Outputs=3
  Selector : Selector  InputPortWidth=3  IndexOptions=Index vector (dialog)  Indices=[1]  OutputSizes=1
  Selector1 : Selector  InputPortWidth=3  IndexOptions=Index vector (dialog)  Indices=[2]  OutputSizes=1
  States : Outport
  wires:
  Demux/2 -> Bus Creator/2  "y"
  UAVState/1 -> Bus Selector/1
  Bus Selector/2 -> Selector/1, Selector1/1  "<Ve>"
  Bus Selector/1 -> Demux/1  "<Xe>"
  Demux/1 -> Bus Creator/1  "x"
  Selector/1 -> Bus Creator/4  "vx"
  Demux/3 -> Bus Creator/3  "z"
  Selector1/1 -> Bus Creator/5  "vy"
  Bus Creator/1 -> States/1

== system VTOLAutopilotController/Guidance Test Bench/ControlType/Guidance Testbench/Guidance Logic/Subsystem ==
  note: Tilt Angle also determines the state aircraft is in. Thus a unit delay is added
  UAVState : Inport
  Bus Creator : BusCreator  Inputs=6  OutDataTypeStr=Bus: GuidanceStates
  Bus Selector : BusSelector  OutputSignals=Euler,pqr,Ve,Xe,course,RotorParameters.Tilt1,airspeed
  Gain : Gain
  Unit Delay : UnitDelay  InitialCondition=tiltIni  SampleTime=-1  HasFrameUpgradeWarning=on
  States : Outport
  wires:
  UAVState/1 -> Bus Selector/1
  Bus Selector/1 -> Bus Creator/1  "<Euler>"
  Bus Creator/1 -> States/1
  Bus Selector/3 -> Bus Creator/3  "<Ve>"
  Bus Selector/2 -> Bus Creator/2  "<pqr>"
  Bus Selector/4 -> Bus Creator/4  "<Xe>"
  Bus Selector/5 -> Bus Creator/5  "<course>"
  Gain/1 -> Bus Creator/6  "Tilt"
  Unit Delay/1 -> Gain/1  "Tilt1"
  Bus Selector/6 -> Unit Delay/1  "<Tilt1>"

== system VTOLAutopilotController/Guidance Test Bench/ControlType/Manual Control/Command Interface/Control Rate Transition ==
  FM : Inport
  "ControlMode " : Inport  Port=2
  FixedWingSetpoint : Inport  Port=3
  AACSetpoint : Inport  Port=4
  Position : Inport  Port=5
  Rate Transition{,1..3,5} (5 alike) : RateTransition  OutPortSampleTime=ControlSampleTime
  ctrlMode : Outport
  FixedWingSP : Outport  Port=2
  AACSP : Outport  Port=3
  PositionCmds : Outport  Port=4
  FlightMode : Outport  Port=5
  wires:
  Rate Transition5/1 -> FlightMode/1
  Position/1 -> Rate Transition3/1
  FixedWingSetpoint/1 -> Rate Transition1/1
  Rate Transition3/1 -> PositionCmds/1
  FM/1 -> Rate Transition5/1
  "ControlMode "/1 -> Rate Transition/1
  Rate Transition1/1 -> FixedWingSP/1
  AACSetpoint/1 -> Rate Transition2/1
  Rate Transition2/1 -> AACSP/1
  Rate Transition/1 -> ctrlMode/1

== system VTOLAutopilotController/Guidance Test Bench/ControlType/Manual Control/Command Interface/Subsystem ==
  note: Tilt Angle also determines the state aircraft is in. Thus a unit delay is added
  UAVState : Inport
  Bus Creator : BusCreator  Inputs=6  OutDataTypeStr=Bus: GuidanceStates
  Bus Selector : BusSelector  OutputSignals=Euler,pqr,Ve,Xe,course,RotorParameters.Tilt1
  Gain : Gain
  Unit Delay : UnitDelay  InitialCondition=tiltIni  SampleTime=-1  HasFrameUpgradeWarning=on
  States : Outport
  wires:
  UAVState/1 -> Bus Selector/1
  Bus Selector/1 -> Bus Creator/1  "<Euler>"
  Bus Creator/1 -> States/1
  Bus Selector/3 -> Bus Creator/3  "<Ve>"
  Bus Selector/2 -> Bus Creator/2  "<pqr>"
  Bus Selector/4 -> Bus Creator/4  "<Xe>"
  Bus Selector/5 -> Bus Creator/5  "<course>"
  Bus Selector/6 -> Unit Delay/1  "<Tilt1>"
  Gain/1 -> Bus Creator/6  "Tilt"
  Unit Delay/1 -> Gain/1  "Tilt2"

== system VTOLAutopilotController/Low level controller/Fixed Wing Controller/Fixed Wing Controller Module/Fixed Wing Controller Simulation/AER from Path Manager ==
  In1 : Inport
  Enable : EnablePort
  Out1 : Outport
  wires:
  In1/1 -> Out1/1

== system VTOLAutopilotController/Low level controller/Fixed Wing Controller/Fixed Wing Controller Module/Fixed Wing Controller Simulation/Airspeed-Altitude Controller ==
  note: Airspeed and altitude are controlled independently
      | by ignoring their coupled dynamics.
  Airspeed SP : Inport
  Altitude SP : Inport  Port=2
  Climb Rate SP : Inport  Port=3
  Airspeed : Inport  Port=4
  xyz : Inport  Port=5
  vxyz : Inport  Port=6
  Flight Mode : Inport  Port=7
  Enable : EnablePort  ShowOutputPort=on
  Airspeed Controller : slpidlib/PID Controller  Controller=PID  Form=Parallel  TimeDomain=Discrete-time  UseExternalTs=off  SampleTime=-1  IntegratorMethod=Trapezoidal  FilterMethod=Forward Euler  ControllerParametersSource=internal  P=FWControlParams.P_AIRSPD  I=FWControlParams.I_AIRSPD  UseKiTs=off  D=FWControlParams.D_AIRSPD  UseExternalDerivativeSource=off  N=FWControlParams.N_AIRSPD  UseFilter=on  TunerSelectOption=Transfer Function Based (PID Tuner App)  InitialConditionSource=external  InitialConditionForIntegrator=0  InitialConditionForFilter=0  DifferentiatorICPrevScaledInput=0  ExternalReset=level  TrackingMode=off  Kt=1  LimitOutput=off  SatLimitsSource=internal  UpperSaturationLimit=Inf  LowerSaturationLimit=0  LinearizeAsGain=on  AntiWindupMode=clamping  Kb=1  LimitIntegrator=off  UpperIntegratorSaturationLimit=inf  LowerIntegratorSaturationLimit=-inf  POutMin=[]  POutMax=[]  IOutMin=[]  IOutMax=[]  DOutMin=[]  DOutMax=[]  NOutMin=[]  NOutMax=[]  SumOutMin=[]  SumOutMax=[]  SaturationOutMin=[]  SaturationOutMax=[]  PParamMin=[]  PParamMax=[]  IParamMin=[]  IParamMax=[]  DParamMin=[]  DParamMax=[]  NParamMin=[]  NParamMax=[]  KbParamMin=[]  KbParamMax=[]  KtParamMin=[]  KtParamMax=[]  KbOutMin=[]  KbOutMax=[]  KtOutMin=[]  KtOutMax=[]  IntegratorOutMin=[]  IntegratorOutMax=[]  FilterOutMin=[]  FilterOutMax=[]  SumI1OutMin=[]  SumI1OutMax=[]  SumI2OutMin=[]  SumI2OutMax=[]  SumI3OutMin=[]  SumI3OutMax=[]  SumI4OutMin=[]  SumI4OutMax=[]  SumDOutMin=[]  SumDOutMax=[]  DifferentiatorOutMin=[]  DifferentiatorOutMax=[]  FilterDiffOutCoefMin=[]  FilterDiffOutCoefMax=[]  ReciprocalOutMin=[]  ReciprocalOutMax=[]  SumDenOutMin=[]  SumDenOutMax=[]  SumNumOutMin=[]  SumNumOutMax=[]  DivideOutMin=[]  DivideOutMax=[]  UdiffTsProdOutMin=[]  UdiffTsProdOutMax=[]  NTsProdOutMin=[]  NTsProdOutMax=[]  UintegralTsProdOutMin=[]  UintegralTsProdOutMax=[]  UngainTsProdOutMin=[]  UngainTsProdOutMax=[]  ClampingZeroOutDataTypeStr=Inherit: Inherit via back propagation  ClampingZeroOutMin=[]  ClampingZeroOutMax=[]  FilterDenConstantOutDataTypeStr=Inherit: Inherit via back propagation  FilterDenConstantOutMin=[]  FilterDenConstantOutMax=[]  PCopyOutDataTypeStr=Inherit: Inherit via back propagation  PCopyOutMin=[]  PCopyOutMax=[]  NCopyOutDataTypeStr=Inherit: Inherit via back propagation  NCopyOutMin=[]  NCopyOutMax=[]  IntegratorContinuousStateAttributes=''  IntegratorStateMustResolveToSignalObject=off  IntegratorRTWStateStorageClass=Auto  FilterContinuousStateAttributes=''  FilterStateMustResolveToSignalObject=off  FilterRTWStateStorageClass=Auto  ParallelPVariant=InternalParameters  IdealPVariant=Disabled  IVariant=InternalParameters  DVariant=InternalParameters  IntegratorVariant=Discrete  SatVariant=Disabled  AWVariant=Passthrough  PCopyVariant=Disabled  TRVariant=Disabled  FdbkBlocksVariant=Forward  IdealPFdbkVariant=Disabled  SatFdbkVariant=Disabled  DerivativeFilterVariant=ForwardEulerFilter  NVariant=InternalParameters  NCopyVariant=Disabled  FilterICVariant=ExternalICs  IntegratorICVariant=ExternalICs  ExternalResetVariant=ExternalReset  TRSumVariant=Passthrough  SumFdbkVariant=Disabled  SumVariant=Sum_PID  TsampFilterVariant=InternalTs  TsampNgainVariant=Passthrough  TsampIntegralVariant=Disabled_SignalSpec  ExternalSaturationOutDataTypeStr=Inherit: Same as second input  DerivativeSourceVariant=ErrorSignal  PreIntVariant=InternalPreInt
  Altitude controller : Subsystem
  Climb Rate SP Merge : Merge
  Climb Rate SP from Guidance : Subsystem  TreatAsAtomicUnit=on
  Compare To Constant : simulink/Logic and Bit Operations/Compare To Constant  relop===  const=uint8(1)  OutDataTypeStr=boolean
  Compare To Constant1 : simulink/Logic and Bit Operations/Compare To Constant  relop===  const=uint8(2)  OutDataTypeStr=boolean
  Constant : Constant  Value=flightState.Hover
  Constant1 : Constant  Value=0
  Constant2 : Constant  Value=flightState.Transition
  Constant5 : Constant  Value=controlParams.FWTrimThrottle
  Equal : RelationalOperator  Operator===  OutDataTypeStr=boolean  RndMeth=Simplest  InputSameDT=off
  Equal1 : RelationalOperator  Operator===  OutDataTypeStr=boolean  RndMeth=Simplest  InputSameDT=off
  Gain7 : Gain  Gain=controlParams.VTOLthrCoefficient
  Logical Operator : Logic  Operator=OR  AllPortsSameDT=off  OutDataTypeStr=boolean
  Mux : Mux  Inputs=2
  Pitch SP Controller : Subsystem
  Rate Limiter : RateLimiter  RisingSlewLimit=controlParams.FWmaxpitchCMDratelimit  FallingSlewLimit=controlParams.FWminpitchCMDratelimit  SampleTimeMode=inherited
  Scope : Scope
      settings: ActiveDisplayYMinimum=32.8352  ActiveDisplayYMaximum=39.52044  DataLoggingVariableName=ScopeData3
  Square : Math  Operator=square
  Sum1 : Sum  Inputs=|+-
  Pitch SP : Outport
  Throttle : Outport  Port=2
  wires:
  Airspeed SP/1 -> Mux/1, Sum1/1
  Sum1/1 -> Airspeed Controller/1
  Airspeed/1 -> Mux/2, Sum1/2
  Airspeed Controller/1 -> Throttle/1
  Altitude SP/1 -> Altitude controller/1(Alt SP)
  xyz/1 -> Altitude controller/2(xyz)
  vxyz/1 -> Pitch SP Controller/2(vxyz)
  Pitch SP Controller/1(Pitch SP) -> Rate Limiter/1
  Enable/1 -> Compare To Constant/1, Compare To Constant1/1
  Compare To Constant/1 -> Altitude controller/Enable
  Compare To Constant1/1 -> Climb Rate SP from Guidance/Enable
  Altitude controller/1(Climb Rate SP) -> Climb Rate SP Merge/1
  Climb Rate SP from Guidance/1(Out1) -> Climb Rate SP Merge/2
  Climb Rate SP Merge/1 -> Pitch SP Controller/1(Climb Rate SP)
  Climb Rate SP/1 -> Climb Rate SP from Guidance/1(Climb Rate SP)
  Rate Limiter/1 -> Pitch SP/1
  Flight Mode/1 -> [FlightMode]
  [FlightMode] -> Pitch SP Controller/3(Flight Mode)
  [int_thr_reset] -> Airspeed Controller/2
  Constant1/1 -> Airspeed Controller/4
  Constant5/1 -> Square/1
  Square/1 -> Gain7/1
  Gain7/1 -> Airspeed Controller/3
  Mux/1 -> Scope/1
  Constant/1 -> Equal/2
  [FlightMode] -> Equal/1
  Constant2/1 -> Equal1/2
  [FlightMode] -> Equal1/1
  Equal1/1 -> Logical Operator/2
  Equal/1 -> Logical Operator/1
  Logical Operator/1 -> [int_thr_reset]

== system VTOLAutopilotController/Low level controller/Fixed Wing Controller/Fixed Wing Controller Module/Fixed Wing Controller Simulation/Attitude Controller ==
  YPR SP : Inport
  ypr : Inport  Port=2
  EulRate : Inport  Port=3
  Airspeed : Inport  Port=4
  AoS : Inport  Port=5
  Flight Mode : Inport  Port=6
  Enable : EnablePort  ShowOutputPort=on
  AER Merge : Merge
  Compare To Constant : simulink/Logic and Bit Operations/Compare To Constant  relop===  const=uint8(1)  OutDataTypeStr=boolean
  Compare To Constant1 : simulink/Logic and Bit Operations/Compare To Constant  relop===  const=uint8(2)  OutDataTypeStr=boolean
  Demux1 : Demux  Outputs=3
  Pitch Roll Controller : Subsystem
  Rudder Heading Controller : Subsystem
  AER : Outport
  wires:
  YPR SP/1 -> Demux1/1
  Enable/1 -> Compare To Constant1/1, Compare To Constant/1
  AER Merge/1 -> AER/1
  Compare To Constant/1 -> Pitch Roll Controller/Enable
  Pitch Roll Controller/1(AER) -> AER Merge/1
  Rudder Heading Controller/1(AER) -> AER Merge/2
  [Roll_SP] -> Pitch Roll Controller/2(Roll SP)
  Compare To Constant1/1 -> Rudder Heading Controller/Enable
  Demux1/1 -> [Yaw_SP]
  Demux1/2 -> [Pitch_SP]
  Demux1/3 -> [Roll_SP]
  [Pitch_SP] -> Pitch Roll Controller/1(Pitch SP)
  Airspeed/1 -> [Air_SPD]
  EulRate/1 -> [EulerRate]
  [EulerRate] -> Pitch Roll Controller/4(EulerRate)
  [Air_SPD] -> Pitch Roll Controller/5(Airspeed)
  ypr/1 -> [YPR]
  [YPR] -> Pitch Roll Controller/3(YPR)
  [Yaw_SP] -> Rudder Heading Controller/1(Yaw SP)
  [YPR] -> Rudder Heading Controller/2(YPR)
  [EulerRate] -> Rudder Heading Controller/3(Ang Rate)
  AoS/1 -> [AoS]
  [AoS] -> Pitch Roll Controller/6(AoS)
  Flight Mode/1 -> Pitch Roll Controller/7(Flight Mode)

== system VTOLAutopilotController/Low level controller/Fixed Wing Controller/Fixed Wing Controller Module/Fixed Wing Controller Simulation/Lateral Guidance Logic ==
  note: S. Park, J. Deyst, and J. P. How, "A New Nonlinear Guidance Logic for Trajectory Tracking," Proceedings of the AIAA Guidance, Navigation and Control Conference, Aug 2004. AIAA-2004-4900.
  Course SP : Inport
  L1 Distance : Inport  Port=2
  course : Inport  Port=3
  gndspeed : Inport  Port=4
  Enable : EnablePort
  MATLAB Function : MATLAB Function  TreatAsAtomicUnit=on
  Terminator : Terminator
  Roll SP : Outport
  wires:
  Course SP/1 -> MATLAB Function/1(courseSP)
  course/1 -> MATLAB Function/2(course)
  MATLAB Function/2(rollSP) -> Roll SP/1
  MATLAB Function/1(lacc) -> Terminator/1
  gndspeed/1 -> MATLAB Function/3(groundSpeed)
  L1 Distance/1 -> MATLAB Function/4(L1)

== system VTOLAutopilotController/Low level controller/Fixed Wing Controller/Fixed Wing Controller Module/Fixed Wing Controller Simulation/Pitch, Airspeed SP from Controller ==
  Pitch SP In : Inport
  Airspeed SP : Inport  Port=2
  Airspeed : Inport  Port=3
  Enable : EnablePort
  Airspeed Controller : slpidlib/PID Controller  Controller=PID  Form=Parallel  TimeDomain=Discrete-time  UseExternalTs=off  SampleTime=-1  IntegratorMethod=Trapezoidal  FilterMethod=Forward Euler  ControllerParametersSource=internal  P=FWControlParams.P_AIRSPD  I=FWControlParams.I_AIRSPD*0  UseKiTs=off  D=FWControlParams.D_AIRSPD*0  UseExternalDerivativeSource=off  N=FWControlParams.N_AIRSPD  UseFilter=on  TunerSelectOption=Transfer Function Based (PID Tuner App)  InitialConditionSource=internal  InitialConditionForIntegrator=0  InitialConditionForFilter=0  DifferentiatorICPrevScaledInput=0  ExternalReset=none  TrackingMode=off  Kt=1  LimitOutput=off  SatLimitsSource=internal  UpperSaturationLimit=Inf  LowerSaturationLimit=0  LinearizeAsGain=on  AntiWindupMode=clamping  Kb=1  LimitIntegrator=off  UpperIntegratorSaturationLimit=inf  LowerIntegratorSaturationLimit=-inf  POutMin=[]  POutMax=[]  IOutMin=[]  IOutMax=[]  DOutMin=[]  DOutMax=[]  NOutMin=[]  NOutMax=[]  SumOutMin=[]  SumOutMax=[]  SaturationOutMin=[]  SaturationOutMax=[]  PParamMin=[]  PParamMax=[]  IParamMin=[]  IParamMax=[]  DParamMin=[]  DParamMax=[]  NParamMin=[]  NParamMax=[]  KbParamMin=[]  KbParamMax=[]  KtParamMin=[]  KtParamMax=[]  KbOutMin=[]  KbOutMax=[]  KtOutMin=[]  KtOutMax=[]  IntegratorOutMin=[]  IntegratorOutMax=[]  FilterOutMin=[]  FilterOutMax=[]  SumI1OutMin=[]  SumI1OutMax=[]  SumI2OutMin=[]  SumI2OutMax=[]  SumI3OutMin=[]  SumI3OutMax=[]  SumI4OutMin=[]  SumI4OutMax=[]  SumDOutMin=[]  SumDOutMax=[]  DifferentiatorOutMin=[]  DifferentiatorOutMax=[]  FilterDiffOutCoefMin=[]  FilterDiffOutCoefMax=[]  ReciprocalOutMin=[]  ReciprocalOutMax=[]  SumDenOutMin=[]  SumDenOutMax=[]  SumNumOutMin=[]  SumNumOutMax=[]  DivideOutMin=[]  DivideOutMax=[]  UdiffTsProdOutMin=[]  UdiffTsProdOutMax=[]  NTsProdOutMin=[]  NTsProdOutMax=[]  UintegralTsProdOutMin=[]  UintegralTsProdOutMax=[]  UngainTsProdOutMin=[]  UngainTsProdOutMax=[]  ClampingZeroOutDataTypeStr=Inherit: Inherit via back propagation  ClampingZeroOutMin=[]  ClampingZeroOutMax=[]  FilterDenConstantOutDataTypeStr=Inherit: Inherit via back propagation  FilterDenConstantOutMin=[]  FilterDenConstantOutMax=[]  PCopyOutDataTypeStr=Inherit: Inherit via back propagation  PCopyOutMin=[]  PCopyOutMax=[]  NCopyOutDataTypeStr=Inherit: Inherit via back propagation  NCopyOutMin=[]  NCopyOutMax=[]  IntegratorContinuousStateAttributes=''  IntegratorStateMustResolveToSignalObject=off  IntegratorRTWStateStorageClass=Auto  FilterContinuousStateAttributes=''  FilterStateMustResolveToSignalObject=off  FilterRTWStateStorageClass=Auto  ParallelPVariant=InternalParameters  IdealPVariant=Disabled  IVariant=InternalParameters  DVariant=InternalParameters  IntegratorVariant=Discrete  SatVariant=Disabled  AWVariant=Passthrough  PCopyVariant=Disabled  TRVariant=Disabled  FdbkBlocksVariant=Forward  IdealPFdbkVariant=Disabled  SatFdbkVariant=Disabled  DerivativeFilterVariant=ForwardEulerFilter  NVariant=InternalParameters  NCopyVariant=Disabled  FilterICVariant=InternalICsFilter  IntegratorICVariant=InternalICs  ExternalResetVariant=Disabled  TRSumVariant=Passthrough  SumFdbkVariant=Disabled  SumVariant=Sum_PID  TsampFilterVariant=InternalTs  TsampNgainVariant=Passthrough  TsampIntegralVariant=Disabled_SignalSpec  ExternalSaturationOutDataTypeStr=Inherit: Same as second input  DerivativeSourceVariant=ErrorSignal  PreIntVariant=InternalPreInt
  IC : InitialCondition  Value=0
  Sum1 : Sum  Inputs=|+-
  Pitch SP : Outport
  Throttle : Outport  Port=2
  wires:
  IC/1 -> Pitch SP/1
  Pitch SP In/1 -> IC/1
  Airspeed SP/1 -> Sum1/1
  Sum1/1 -> Airspeed Controller/1
  Airspeed/1 -> Sum1/2
  Airspeed Controller/1 -> Throttle/1

== system VTOLAutopilotController/Low level controller/Fixed Wing Controller/Fixed Wing Controller Module/Fixed Wing Controller Simulation/Roll SP from Path Manager ==
  In1 : Inport
  Enable : EnablePort
  IC : InitialCondition  Value=0
  Out1 : Outport
  wires:
  In1/1 -> IC/1
  IC/1 -> Out1/1

== system VTOLAutopilotController/Low level controller/Fixed Wing Controller/Fixed Wing Controller Module/Fixed Wing Controller Simulation/Subsystem2 ==
  Euler : Inport
  pqr : Inport  Port=2
  Demux : Demux  Outputs=3
  MATLAB Function : MATLAB Function  TreatAsAtomicUnit=on
  Terminator : Terminator
  Terminator1 : Terminator
  Euler Rate : Outport
  wires:
  Demux/1 -> MATLAB Function/1(phi)
  Demux/2 -> MATLAB Function/2(theta)
  MATLAB Function/1(y) -> Terminator1/1
  pqr/1 -> Euler Rate/1
  Euler/1 -> Demux/1
  Demux/3 -> Terminator/1

== system VTOLAutopilotController/Low level controller/Fixed Wing Controller/Fixed Wing Controller Module/Fixed Wing Controller Simulation/Visualization ==
  YawSetPoint : Inport
  RollSetPoint : Inport  Port=2
  PitchSetPoint : Inport  Port=3
  YPR : Inport  Port=4
  AirspeedSetPoint : Inport  Port=5
  Airspeed : Inport  Port=6
  AltitudeSetPoint : Inport  Port=7
  XYZ : Inport  Port=8
  No-op : Subsystem  VariantControl=Deployment == true
  Visualization : Subsystem  VariantControl=Deployment == false

== system VTOLAutopilotController/Low level controller/Fixed Wing Controller/Fixed Wing Controller Module/Fixed Wing Controller Tuning/AER from Path Manager ==
  In1 : Inport
  Enable : EnablePort
  Out1 : Outport
  wires:
  In1/1 -> Out1/1
